simulink model "Ground"  (R2015a)
settings: configuration reference "GlobalConfig" (kept outside this file)
PreLoadFcn:
  | modelPreLoadClbck
InitFcn:
  | modelPreLoadClbck
model workspace (MAT data in the model file):
  MCOS : class17 (value not decoded)
libraries: fl_lib x427, nesl_utility x145
(part 4 of 5)

== system Ground/Ground Model 1/GroundUnit45 ==
  Conductive Heat Transfer1 : fl_lib/Thermal/Thermal Elements/Conductive Heat Transfer  area=Area m^2  thickness=Thickness/100 m  th_cond=ThermalConductivity W/(m*K)  Q_specify=off  Q_priority=High  Q=0 J/s  T_specify=off  T_priority=High  T=0 K
      settings: AttributesFormatString=|
      | Area:%<area>
      | ThCond:%<th_cond>
      | Thickness:%<thickness>
  Conductive Heat Transfer2 : fl_lib/Thermal/Thermal Elements/Conductive Heat Transfer  area=Area m^2  thickness=Thickness/100 m  th_cond=ThermalConductivity W/(m*K)  Q_specify=off  Q_priority=High  Q=0 J/s  T_specify=off  T_priority=High  T=0 K
      settings: AttributesFormatString=|
      | Area:%<area>
      | ThCond:%<th_cond>
      | Thickness:%<thickness>
  Ideal Heat Flow Sensor : fl_lib/Thermal/Thermal Sensors/Ideal Heat Flow Sensor
  Ideal Temperature Sensor : fl_lib/Thermal/Thermal Sensors/Ideal Temperature Sensor
  PS-Simulink Converter : nesl_utility/PS-Simulink Converter  PhysicalDomain=network_engine_domain  SubClassName=ps_output  LeftPortType=input  RightPortType=output  PseudoPeriodic=off  Frequencies=[]  Unit=K  AffineConversion=off
  PS-Simulink Converter1 : nesl_utility/PS-Simulink Converter  PhysicalDomain=network_engine_domain  SubClassName=ps_output  LeftPortType=input  RightPortType=output  PseudoPeriodic=off  Frequencies=[]  Unit=J/s  AffineConversion=off
  Thermal Mass : fl_lib/Thermal/Thermal Elements/Thermal Mass  mass=Density*Area*Thickness kg  sp_heat=SpecificHeat J/kg/K  Q_specify=off  Q_priority=High  Q=0 J/s  T_specify=on  T_priority=High  T=Temperature K
      settings: AttributesFormatString=|
      | %<mass>
      | %<sp_heat>
      | %<T>
  Thermal Reference1 : fl_lib/Thermal/Thermal Elements/Thermal Reference
  In : PMIOPort  Port=1  Side=Left
  Out : PMIOPort  Port=2  Side=Left
  Temperature : Outport
  Heat Flow : Outport  Port=2
  wires:
  PS-Simulink Converter/1 -> Temperature/1
  PS-Simulink Converter1/1 -> Heat Flow/1
  connections:
  Conductive Heat Transfer2/RConn1 -- Out/RConn1
  Ideal Temperature Sensor/RConn1 -- Thermal Reference1/LConn1
  Conductive Heat Transfer2/LConn1 -- Ideal Heat Flow Sensor/RConn2
  PS-Simulink Converter/LConn1 -- Ideal Temperature Sensor/RConn2
  In/RConn1 -- Conductive Heat Transfer1/LConn1
  Conductive Heat Transfer1/RConn1 -- Ideal Temperature Sensor/LConn1 -- Ideal Heat Flow Sensor/LConn1 -- Thermal Mass/LConn1
  Ideal Heat Flow Sensor/RConn1 -- PS-Simulink Converter1/LConn1

== system Ground/Ground Model 1/GroundUnit46 ==
  Conductive Heat Transfer1 : fl_lib/Thermal/Thermal Elements/Conductive Heat Transfer  area=Area m^2  thickness=Thickness/100 m  th_cond=ThermalConductivity W/(m*K)  Q_specify=off  Q_priority=High  Q=0 J/s  T_specify=off  T_priority=High  T=0 K
      settings: AttributesFormatString=|
      | Area:%<area>
      | ThCond:%<th_cond>
      | Thickness:%<thickness>
  Conductive Heat Transfer2 : fl_lib/Thermal/Thermal Elements/Conductive Heat Transfer  area=Area m^2  thickness=Thickness/100 m  th_cond=ThermalConductivity W/(m*K)  Q_specify=off  Q_priority=High  Q=0 J/s  T_specify=off  T_priority=High  T=0 K
      settings: AttributesFormatString=|
      | Area:%<area>
      | ThCond:%<th_cond>
      | Thickness:%<thickness>
  Ideal Heat Flow Sensor : fl_lib/Thermal/Thermal Sensors/Ideal Heat Flow Sensor
  Ideal Temperature Sensor : fl_lib/Thermal/Thermal Sensors/Ideal Temperature Sensor
  PS-Simulink Converter : nesl_utility/PS-Simulink Converter  PhysicalDomain=network_engine_domain  SubClassName=ps_output  LeftPortType=input  RightPortType=output  PseudoPeriodic=off  Frequencies=[]  Unit=K  AffineConversion=off
  PS-Simulink Converter1 : nesl_utility/PS-Simulink Converter  PhysicalDomain=network_engine_domain  SubClassName=ps_output  LeftPortType=input  RightPortType=output  PseudoPeriodic=off  Frequencies=[]  Unit=J/s  AffineConversion=off
  Thermal Mass : fl_lib/Thermal/Thermal Elements/Thermal Mass  mass=Density*Area*Thickness kg  sp_heat=SpecificHeat J/kg/K  Q_specify=off  Q_priority=High  Q=0 J/s  T_specify=on  T_priority=High  T=Temperature K
      settings: AttributesFormatString=|
      | %<mass>
      | %<sp_heat>
      | %<T>
  Thermal Reference1 : fl_lib/Thermal/Thermal Elements/Thermal Reference
  In : PMIOPort  Port=1  Side=Left
  Out : PMIOPort  Port=2  Side=Left
  Temperature : Outport
  Heat Flow : Outport  Port=2
  wires:
  PS-Simulink Converter/1 -> Temperature/1
  PS-Simulink Converter1/1 -> Heat Flow/1
  connections:
  Conductive Heat Transfer2/RConn1 -- Out/RConn1
  Ideal Temperature Sensor/RConn1 -- Thermal Reference1/LConn1
  Conductive Heat Transfer2/LConn1 -- Ideal Heat Flow Sensor/RConn2
  PS-Simulink Converter/LConn1 -- Ideal Temperature Sensor/RConn2
  In/RConn1 -- Conductive Heat Transfer1/LConn1
  Conductive Heat Transfer1/RConn1 -- Ideal Temperature Sensor/LConn1 -- Ideal Heat Flow Sensor/LConn1 -- Thermal Mass/LConn1
  Ideal Heat Flow Sensor/RConn1 -- PS-Simulink Converter1/LConn1

== system Ground/Ground Model 1/GroundUnit47 ==
  Conductive Heat Transfer1 : fl_lib/Thermal/Thermal Elements/Conductive Heat Transfer  area=Area m^2  thickness=Thickness/100 m  th_cond=ThermalConductivity W/(m*K)  Q_specify=off  Q_priority=High  Q=0 J/s  T_specify=off  T_priority=High  T=0 K
      settings: AttributesFormatString=|
      | Area:%<area>
      | ThCond:%<th_cond>
      | Thickness:%<thickness>
  Conductive Heat Transfer2 : fl_lib/Thermal/Thermal Elements/Conductive Heat Transfer  area=Area m^2  thickness=Thickness/100 m  th_cond=ThermalConductivity W/(m*K)  Q_specify=off  Q_priority=High  Q=0 J/s  T_specify=off  T_priority=High  T=0 K
      settings: AttributesFormatString=|
      | Area:%<area>
      | ThCond:%<th_cond>
      | Thickness:%<thickness>
  Ideal Heat Flow Sensor : fl_lib/Thermal/Thermal Sensors/Ideal Heat Flow Sensor
  Ideal Temperature Sensor : fl_lib/Thermal/Thermal Sensors/Ideal Temperature Sensor
  PS-Simulink Converter : nesl_utility/PS-Simulink Converter  PhysicalDomain=network_engine_domain  SubClassName=ps_output  LeftPortType=input  RightPortType=output  PseudoPeriodic=off  Frequencies=[]  Unit=K  AffineConversion=off
  PS-Simulink Converter1 : nesl_utility/PS-Simulink Converter  PhysicalDomain=network_engine_domain  SubClassName=ps_output  LeftPortType=input  RightPortType=output  PseudoPeriodic=off  Frequencies=[]  Unit=J/s  AffineConversion=off
  Thermal Mass : fl_lib/Thermal/Thermal Elements/Thermal Mass  mass=Density*Area*Thickness kg  sp_heat=SpecificHeat J/kg/K  Q_specify=off  Q_priority=High  Q=0 J/s  T_specify=on  T_priority=High  T=Temperature K
      settings: AttributesFormatString=|
      | %<mass>
      | %<sp_heat>
      | %<T>
  Thermal Reference1 : fl_lib/Thermal/Thermal Elements/Thermal Reference
  In : PMIOPort  Port=1  Side=Left
  Out : PMIOPort  Port=2  Side=Left
  Temperature : Outport
  Heat Flow : Outport  Port=2
  wires:
  PS-Simulink Converter/1 -> Temperature/1
  PS-Simulink Converter1/1 -> Heat Flow/1
  connections:
  Conductive Heat Transfer2/RConn1 -- Out/RConn1
  Ideal Temperature Sensor/RConn1 -- Thermal Reference1/LConn1
  Conductive Heat Transfer2/LConn1 -- Ideal Heat Flow Sensor/RConn2
  PS-Simulink Converter/LConn1 -- Ideal Temperature Sensor/RConn2
  In/RConn1 -- Conductive Heat Transfer1/LConn1
  Conductive Heat Transfer1/RConn1 -- Ideal Temperature Sensor/LConn1 -- Ideal Heat Flow Sensor/LConn1 -- Thermal Mass/LConn1
  Ideal Heat Flow Sensor/RConn1 -- PS-Simulink Converter1/LConn1

== system Ground/Ground Model 1/GroundUnit48 ==
  Conductive Heat Transfer1 : fl_lib/Thermal/Thermal Elements/Conductive Heat Transfer  area=Area m^2  thickness=Thickness/100 m  th_cond=ThermalConductivity W/(m*K)  Q_specify=off  Q_priority=High  Q=0 J/s  T_specify=off  T_priority=High  T=0 K
      settings: AttributesFormatString=|
      | Area:%<area>
      | ThCond:%<th_cond>
      | Thickness:%<thickness>
  Conductive Heat Transfer2 : fl_lib/Thermal/Thermal Elements/Conductive Heat Transfer  area=Area m^2  thickness=Thickness/100 m  th_cond=ThermalConductivity W/(m*K)  Q_specify=off  Q_priority=High  Q=0 J/s  T_specify=off  T_priority=High  T=0 K
      settings: AttributesFormatString=|
      | Area:%<area>
      | ThCond:%<th_cond>
      | Thickness:%<thickness>
  Ideal Heat Flow Sensor : fl_lib/Thermal/Thermal Sensors/Ideal Heat Flow Sensor
  Ideal Temperature Sensor : fl_lib/Thermal/Thermal Sensors/Ideal Temperature Sensor
  PS-Simulink Converter : nesl_utility/PS-Simulink Converter  PhysicalDomain=network_engine_domain  SubClassName=ps_output  LeftPortType=input  RightPortType=output  PseudoPeriodic=off  Frequencies=[]  Unit=K  AffineConversion=off
  PS-Simulink Converter1 : nesl_utility/PS-Simulink Converter  PhysicalDomain=network_engine_domain  SubClassName=ps_output  LeftPortType=input  RightPortType=output  PseudoPeriodic=off  Frequencies=[]  Unit=J/s  AffineConversion=off
  Thermal Mass : fl_lib/Thermal/Thermal Elements/Thermal Mass  mass=Density*Area*Thickness kg  sp_heat=SpecificHeat J/kg/K  Q_specify=off  Q_priority=High  Q=0 J/s  T_specify=on  T_priority=High  T=Temperature K
      settings: AttributesFormatString=|
      | %<mass>
      | %<sp_heat>
      | %<T>
  Thermal Reference1 : fl_lib/Thermal/Thermal Elements/Thermal Reference
  In : PMIOPort  Port=1  Side=Left
  Out : PMIOPort  Port=2  Side=Left
  Temperature : Outport
  Heat Flow : Outport  Port=2
  wires:
  PS-Simulink Converter/1 -> Temperature/1
  PS-Simulink Converter1/1 -> Heat Flow/1
  connections:
  Conductive Heat Transfer2/RConn1 -- Out/RConn1
  Ideal Temperature Sensor/RConn1 -- Thermal Reference1/LConn1
  Conductive Heat Transfer2/LConn1 -- Ideal Heat Flow Sensor/RConn2
  PS-Simulink Converter/LConn1 -- Ideal Temperature Sensor/RConn2
  In/RConn1 -- Conductive Heat Transfer1/LConn1
  Conductive Heat Transfer1/RConn1 -- Ideal Temperature Sensor/LConn1 -- Ideal Heat Flow Sensor/LConn1 -- Thermal Mass/LConn1
  Ideal Heat Flow Sensor/RConn1 -- PS-Simulink Converter1/LConn1

== system Ground/Ground Model 1/GroundUnit49 ==
  Conductive Heat Transfer1 : fl_lib/Thermal/Thermal Elements/Conductive Heat Transfer  area=Area m^2  thickness=Thickness/100 m  th_cond=ThermalConductivity W/(m*K)  Q_specify=off  Q_priority=High  Q=0 J/s  T_specify=off  T_priority=High  T=0 K
      settings: AttributesFormatString=|
      | Area:%<area>
      | ThCond:%<th_cond>
      | Thickness:%<thickness>
  Conductive Heat Transfer2 : fl_lib/Thermal/Thermal Elements/Conductive Heat Transfer  area=Area m^2  thickness=Thickness/100 m  th_cond=ThermalConductivity W/(m*K)  Q_specify=off  Q_priority=High  Q=0 J/s  T_specify=off  T_priority=High  T=0 K
      settings: AttributesFormatString=|
      | Area:%<area>
      | ThCond:%<th_cond>
      | Thickness:%<thickness>
  Ideal Heat Flow Sensor : fl_lib/Thermal/Thermal Sensors/Ideal Heat Flow Sensor
  Ideal Temperature Sensor : fl_lib/Thermal/Thermal Sensors/Ideal Temperature Sensor
  PS-Simulink Converter : nesl_utility/PS-Simulink Converter  PhysicalDomain=network_engine_domain  SubClassName=ps_output  LeftPortType=input  RightPortType=output  PseudoPeriodic=off  Frequencies=[]  Unit=K  AffineConversion=off
  PS-Simulink Converter1 : nesl_utility/PS-Simulink Converter  PhysicalDomain=network_engine_domain  SubClassName=ps_output  LeftPortType=input  RightPortType=output  PseudoPeriodic=off  Frequencies=[]  Unit=J/s  AffineConversion=off
  Thermal Mass : fl_lib/Thermal/Thermal Elements/Thermal Mass  mass=Density*Area*Thickness kg  sp_heat=SpecificHeat J/kg/K  Q_specify=off  Q_priority=High  Q=0 J/s  T_specify=on  T_priority=High  T=Temperature K
      settings: AttributesFormatString=|
      | %<mass>
      | %<sp_heat>
      | %<T>
  Thermal Reference1 : fl_lib/Thermal/Thermal Elements/Thermal Reference
  In : PMIOPort  Port=1  Side=Left
  Out : PMIOPort  Port=2  Side=Left
  Temperature : Outport
  Heat Flow : Outport  Port=2
  wires:
  PS-Simulink Converter/1 -> Temperature/1
  PS-Simulink Converter1/1 -> Heat Flow/1
  connections:
  Conductive Heat Transfer2/RConn1 -- Out/RConn1
  Ideal Temperature Sensor/RConn1 -- Thermal Reference1/LConn1
  Conductive Heat Transfer2/LConn1 -- Ideal Heat Flow Sensor/RConn2
  PS-Simulink Converter/LConn1 -- Ideal Temperature Sensor/RConn2
  In/RConn1 -- Conductive Heat Transfer1/LConn1
  Conductive Heat Transfer1/RConn1 -- Ideal Temperature Sensor/LConn1 -- Ideal Heat Flow Sensor/LConn1 -- Thermal Mass/LConn1
  Ideal Heat Flow Sensor/RConn1 -- PS-Simulink Converter1/LConn1

== system Ground/Ground Model 1/GroundUnit5 ==
  Conductive Heat Transfer1 : fl_lib/Thermal/Thermal Elements/Conductive Heat Transfer  area=Area m^2  thickness=Thickness/100 m  th_cond=ThermalConductivity W/(m*K)  Q_specify=off  Q_priority=High  Q=0 J/s  T_specify=off  T_priority=High  T=0 K
      settings: AttributesFormatString=|
      | Area:%<area>
      | ThCond:%<th_cond>
      | Thickness:%<thickness>
  Conductive Heat Transfer2 : fl_lib/Thermal/Thermal Elements/Conductive Heat Transfer  area=Area m^2  thickness=Thickness/100 m  th_cond=ThermalConductivity W/(m*K)  Q_specify=off  Q_priority=High  Q=0 J/s  T_specify=off  T_priority=High  T=0 K
      settings: AttributesFormatString=|
      | Area:%<area>
      | ThCond:%<th_cond>
      | Thickness:%<thickness>
  Ideal Heat Flow Sensor : fl_lib/Thermal/Thermal Sensors/Ideal Heat Flow Sensor
  Ideal Temperature Sensor : fl_lib/Thermal/Thermal Sensors/Ideal Temperature Sensor
  PS-Simulink Converter : nesl_utility/PS-Simulink Converter  PhysicalDomain=network_engine_domain  SubClassName=ps_output  LeftPortType=input  RightPortType=output  PseudoPeriodic=off  Frequencies=[]  Unit=K  AffineConversion=off
  PS-Simulink Converter1 : nesl_utility/PS-Simulink Converter  PhysicalDomain=network_engine_domain  SubClassName=ps_output  LeftPortType=input  RightPortType=output  PseudoPeriodic=off  Frequencies=[]  Unit=J/s  AffineConversion=off
  Thermal Mass : fl_lib/Thermal/Thermal Elements/Thermal Mass  mass=Density*Area*Thickness kg  sp_heat=SpecificHeat J/kg/K  Q_specify=off  Q_priority=High  Q=0 J/s  T_specify=on  T_priority=High  T=Temperature K
      settings: AttributesFormatString=|
      | %<mass>
      | %<sp_heat>
      | %<T>
  Thermal Reference1 : fl_lib/Thermal/Thermal Elements/Thermal Reference
  In : PMIOPort  Port=1  Side=Left
  Out : PMIOPort  Port=2  Side=Left
  Temperature : Outport
  Heat Flow : Outport  Port=2
  wires:
  PS-Simulink Converter/1 -> Temperature/1
  PS-Simulink Converter1/1 -> Heat Flow/1
  connections:
  Conductive Heat Transfer2/RConn1 -- Out/RConn1
  Ideal Temperature Sensor/RConn1 -- Thermal Reference1/LConn1
  Conductive Heat Transfer2/LConn1 -- Ideal Heat Flow Sensor/RConn2
  PS-Simulink Converter/LConn1 -- Ideal Temperature Sensor/RConn2
  In/RConn1 -- Conductive Heat Transfer1/LConn1
  Conductive Heat Transfer1/RConn1 -- Ideal Temperature Sensor/LConn1 -- Ideal Heat Flow Sensor/LConn1 -- Thermal Mass/LConn1
  Ideal Heat Flow Sensor/RConn1 -- PS-Simulink Converter1/LConn1

== system Ground/Ground Model 1/GroundUnit6 ==
  Conductive Heat Transfer1 : fl_lib/Thermal/Thermal Elements/Conductive Heat Transfer  area=Area m^2  thickness=Thickness/100 m  th_cond=ThermalConductivity W/(m*K)  Q_specify=off  Q_priority=High  Q=0 J/s  T_specify=off  T_priority=High  T=0 K
      settings: AttributesFormatString=|
      | Area:%<area>
      | ThCond:%<th_cond>
      | Thickness:%<thickness>
  Conductive Heat Transfer2 : fl_lib/Thermal/Thermal Elements/Conductive Heat Transfer  area=Area m^2  thickness=Thickness/100 m  th_cond=ThermalConductivity W/(m*K)  Q_specify=off  Q_priority=High  Q=0 J/s  T_specify=off  T_priority=High  T=0 K
      settings: AttributesFormatString=|
      | Area:%<area>
      | ThCond:%<th_cond>
      | Thickness:%<thickness>
  Ideal Heat Flow Sensor : fl_lib/Thermal/Thermal Sensors/Ideal Heat Flow Sensor
  Ideal Temperature Sensor : fl_lib/Thermal/Thermal Sensors/Ideal Temperature Sensor
  PS-Simulink Converter : nesl_utility/PS-Simulink Converter  PhysicalDomain=network_engine_domain  SubClassName=ps_output  LeftPortType=input  RightPortType=output  PseudoPeriodic=off  Frequencies=[]  Unit=K  AffineConversion=off
  PS-Simulink Converter1 : nesl_utility/PS-Simulink Converter  PhysicalDomain=network_engine_domain  SubClassName=ps_output  LeftPortType=input  RightPortType=output  PseudoPeriodic=off  Frequencies=[]  Unit=J/s  AffineConversion=off
  Thermal Mass : fl_lib/Thermal/Thermal Elements/Thermal Mass  mass=Density*Area*Thickness kg  sp_heat=SpecificHeat J/kg/K  Q_specify=off  Q_priority=High  Q=0 J/s  T_specify=on  T_priority=High  T=Temperature K
      settings: AttributesFormatString=|
      | %<mass>
      | %<sp_heat>
      | %<T>
  Thermal Reference1 : fl_lib/Thermal/Thermal Elements/Thermal Reference
  In : PMIOPort  Port=1  Side=Left
  Out : PMIOPort  Port=2  Side=Left
  Temperature : Outport
  Heat Flow : Outport  Port=2
  wires:
  PS-Simulink Converter/1 -> Temperature/1
  PS-Simulink Converter1/1 -> Heat Flow/1
  connections:
  Conductive Heat Transfer2/RConn1 -- Out/RConn1
  Ideal Temperature Sensor/RConn1 -- Thermal Reference1/LConn1
  Conductive Heat Transfer2/LConn1 -- Ideal Heat Flow Sensor/RConn2
  PS-Simulink Converter/LConn1 -- Ideal Temperature Sensor/RConn2
  In/RConn1 -- Conductive Heat Transfer1/LConn1
  Conductive Heat Transfer1/RConn1 -- Ideal Temperature Sensor/LConn1 -- Ideal Heat Flow Sensor/LConn1 -- Thermal Mass/LConn1
  Ideal Heat Flow Sensor/RConn1 -- PS-Simulink Converter1/LConn1

== system Ground/Ground Model 1/GroundUnit7 ==
  Conductive Heat Transfer1 : fl_lib/Thermal/Thermal Elements/Conductive Heat Transfer  area=Area m^2  thickness=Thickness/100 m  th_cond=ThermalConductivity W/(m*K)  Q_specify=off  Q_priority=High  Q=0 J/s  T_specify=off  T_priority=High  T=0 K
      settings: AttributesFormatString=|
      | Area:%<area>
      | ThCond:%<th_cond>
      | Thickness:%<thickness>
  Conductive Heat Transfer2 : fl_lib/Thermal/Thermal Elements/Conductive Heat Transfer  area=Area m^2  thickness=Thickness/100 m  th_cond=ThermalConductivity W/(m*K)  Q_specify=off  Q_priority=High  Q=0 J/s  T_specify=off  T_priority=High  T=0 K
      settings: AttributesFormatString=|
      | Area:%<area>
      | ThCond:%<th_cond>
      | Thickness:%<thickness>
  Ideal Heat Flow Sensor : fl_lib/Thermal/Thermal Sensors/Ideal Heat Flow Sensor
  Ideal Temperature Sensor : fl_lib/Thermal/Thermal Sensors/Ideal Temperature Sensor
  PS-Simulink Converter : nesl_utility/PS-Simulink Converter  PhysicalDomain=network_engine_domain  SubClassName=ps_output  LeftPortType=input  RightPortType=output  PseudoPeriodic=off  Frequencies=[]  Unit=K  AffineConversion=off
  PS-Simulink Converter1 : nesl_utility/PS-Simulink Converter  PhysicalDomain=network_engine_domain  SubClassName=ps_output  LeftPortType=input  RightPortType=output  PseudoPeriodic=off  Frequencies=[]  Unit=J/s  AffineConversion=off
  Thermal Mass : fl_lib/Thermal/Thermal Elements/Thermal Mass  mass=Density*Area*Thickness kg  sp_heat=SpecificHeat J/kg/K  Q_specify=off  Q_priority=High  Q=0 J/s  T_specify=on  T_priority=High  T=Temperature K
      settings: AttributesFormatString=|
      | %<mass>
      | %<sp_heat>
      | %<T>
  Thermal Reference1 : fl_lib/Thermal/Thermal Elements/Thermal Reference
  In : PMIOPort  Port=1  Side=Left
  Out : PMIOPort  Port=2  Side=Left
  Temperature : Outport
  Heat Flow : Outport  Port=2
  wires:
  PS-Simulink Converter/1 -> Temperature/1
  PS-Simulink Converter1/1 -> Heat Flow/1
  connections:
  Conductive Heat Transfer2/RConn1 -- Out/RConn1
  Ideal Temperature Sensor/RConn1 -- Thermal Reference1/LConn1
  Conductive Heat Transfer2/LConn1 -- Ideal Heat Flow Sensor/RConn2
  PS-Simulink Converter/LConn1 -- Ideal Temperature Sensor/RConn2
  In/RConn1 -- Conductive Heat Transfer1/LConn1
  Conductive Heat Transfer1/RConn1 -- Ideal Temperature Sensor/LConn1 -- Ideal Heat Flow Sensor/LConn1 -- Thermal Mass/LConn1
  Ideal Heat Flow Sensor/RConn1 -- PS-Simulink Converter1/LConn1

== system Ground/Ground Model 1/GroundUnit8 ==
  Conductive Heat Transfer1 : fl_lib/Thermal/Thermal Elements/Conductive Heat Transfer  area=Area m^2  thickness=Thickness/100 m  th_cond=ThermalConductivity W/(m*K)  Q_specify=off  Q_priority=High  Q=0 J/s  T_specify=off  T_priority=High  T=0 K
      settings: AttributesFormatString=|
      | Area:%<area>
      | ThCond:%<th_cond>
      | Thickness:%<thickness>
  Conductive Heat Transfer2 : fl_lib/Thermal/Thermal Elements/Conductive Heat Transfer  area=Area m^2  thickness=Thickness/100 m  th_cond=ThermalConductivity W/(m*K)  Q_specify=off  Q_priority=High  Q=0 J/s  T_specify=off  T_priority=High  T=0 K
      settings: AttributesFormatString=|
      | Area:%<area>
      | ThCond:%<th_cond>
      | Thickness:%<thickness>
  Ideal Heat Flow Sensor : fl_lib/Thermal/Thermal Sensors/Ideal Heat Flow Sensor
  Ideal Temperature Sensor : fl_lib/Thermal/Thermal Sensors/Ideal Temperature Sensor
  PS-Simulink Converter : nesl_utility/PS-Simulink Converter  PhysicalDomain=network_engine_domain  SubClassName=ps_output  LeftPortType=input  RightPortType=output  PseudoPeriodic=off  Frequencies=[]  Unit=K  AffineConversion=off
  PS-Simulink Converter1 : nesl_utility/PS-Simulink Converter  PhysicalDomain=network_engine_domain  SubClassName=ps_output  LeftPortType=input  RightPortType=output  PseudoPeriodic=off  Frequencies=[]  Unit=J/s  AffineConversion=off
  Thermal Mass : fl_lib/Thermal/Thermal Elements/Thermal Mass  mass=Density*Area*Thickness kg  sp_heat=SpecificHeat J/kg/K  Q_specify=off  Q_priority=High  Q=0 J/s  T_specify=on  T_priority=High  T=Temperature K
      settings: AttributesFormatString=|
      | %<mass>
      | %<sp_heat>
      | %<T>
  Thermal Reference1 : fl_lib/Thermal/Thermal Elements/Thermal Reference
  In : PMIOPort  Port=1  Side=Left
  Out : PMIOPort  Port=2  Side=Left
  Temperature : Outport
  Heat Flow : Outport  Port=2
  wires:
  PS-Simulink Converter/1 -> Temperature/1
  PS-Simulink Converter1/1 -> Heat Flow/1
  connections:
  Conductive Heat Transfer2/RConn1 -- Out/RConn1
  Ideal Temperature Sensor/RConn1 -- Thermal Reference1/LConn1
  Conductive Heat Transfer2/LConn1 -- Ideal Heat Flow Sensor/RConn2
  PS-Simulink Converter/LConn1 -- Ideal Temperature Sensor/RConn2
  In/RConn1 -- Conductive Heat Transfer1/LConn1
  Conductive Heat Transfer1/RConn1 -- Ideal Temperature Sensor/LConn1 -- Ideal Heat Flow Sensor/LConn1 -- Thermal Mass/LConn1
  Ideal Heat Flow Sensor/RConn1 -- PS-Simulink Converter1/LConn1

== system Ground/Ground Model 1/GroundUnit9 ==
  Conductive Heat Transfer1 : fl_lib/Thermal/Thermal Elements/Conductive Heat Transfer  area=Area m^2  thickness=Thickness/100 m  th_cond=ThermalConductivity W/(m*K)  Q_specify=off  Q_priority=High  Q=0 J/s  T_specify=off  T_priority=High  T=0 K
      settings: AttributesFormatString=|
      | Area:%<area>
      | ThCond:%<th_cond>
      | Thickness:%<thickness>
  Conductive Heat Transfer2 : fl_lib/Thermal/Thermal Elements/Conductive Heat Transfer  area=Area m^2  thickness=Thickness/100 m  th_cond=ThermalConductivity W/(m*K)  Q_specify=off  Q_priority=High  Q=0 J/s  T_specify=off  T_priority=High  T=0 K
      settings: AttributesFormatString=|
      | Area:%<area>
      | ThCond:%<th_cond>
      | Thickness:%<thickness>
  Ideal Heat Flow Sensor : fl_lib/Thermal/Thermal Sensors/Ideal Heat Flow Sensor
  Ideal Temperature Sensor : fl_lib/Thermal/Thermal Sensors/Ideal Temperature Sensor
  PS-Simulink Converter : nesl_utility/PS-Simulink Converter  PhysicalDomain=network_engine_domain  SubClassName=ps_output  LeftPortType=input  RightPortType=output  PseudoPeriodic=off  Frequencies=[]  Unit=K  AffineConversion=off
  PS-Simulink Converter1 : nesl_utility/PS-Simulink Converter  PhysicalDomain=network_engine_domain  SubClassName=ps_output  LeftPortType=input  RightPortType=output  PseudoPeriodic=off  Frequencies=[]  Unit=J/s  AffineConversion=off
  Thermal Mass : fl_lib/Thermal/Thermal Elements/Thermal Mass  mass=Density*Area*Thickness kg  sp_heat=SpecificHeat J/kg/K  Q_specify=off  Q_priority=High  Q=0 J/s  T_specify=on  T_priority=High  T=Temperature K
      settings: AttributesFormatString=|
      | %<mass>
      | %<sp_heat>
      | %<T>
  Thermal Reference1 : fl_lib/Thermal/Thermal Elements/Thermal Reference
  In : PMIOPort  Port=1  Side=Left
  Out : PMIOPort  Port=2  Side=Left
  Temperature : Outport
  Heat Flow : Outport  Port=2
  wires:
  PS-Simulink Converter/1 -> Temperature/1
  PS-Simulink Converter1/1 -> Heat Flow/1
  connections:
  Conductive Heat Transfer2/RConn1 -- Out/RConn1
  Ideal Temperature Sensor/RConn1 -- Thermal Reference1/LConn1
  Conductive Heat Transfer2/LConn1 -- Ideal Heat Flow Sensor/RConn2
  PS-Simulink Converter/LConn1 -- Ideal Temperature Sensor/RConn2
  In/RConn1 -- Conductive Heat Transfer1/LConn1
  Conductive Heat Transfer1/RConn1 -- Ideal Temperature Sensor/LConn1 -- Ideal Heat Flow Sensor/LConn1 -- Thermal Mass/LConn1
  Ideal Heat Flow Sensor/RConn1 -- PS-Simulink Converter1/LConn1

== system Ground/Ground Model 8/GroundUnit0 ==
  Conductive Heat Transfer1 : fl_lib/Thermal/Thermal Elements/Conductive Heat Transfer  area=Area m^2  thickness=Thickness/MeshNum m  th_cond=ThermalConductivity W/(m*K)  Q_specify=off  Q_priority=High  Q=0 J/s  T_specify=off  T_priority=High  T=0 K
      settings: AttributesFormatString=|
      | Area:%<area>
      | ThCond:%<th_cond>
      | Thickness:%<thickness>
  Conductive Heat Transfer2 : fl_lib/Thermal/Thermal Elements/Conductive Heat Transfer  area=Area m^2  thickness=Thickness/MeshNum m  th_cond=ThermalConductivity W/(m*K)  Q_specify=off  Q_priority=High  Q=0 J/s  T_specify=off  T_priority=High  T=0 K
      settings: AttributesFormatString=|
      | Area:%<area>
      | ThCond:%<th_cond>
      | Thickness:%<thickness>
  Ideal Heat Flow Sensor : fl_lib/Thermal/Thermal Sensors/Ideal Heat Flow Sensor
  Ideal Temperature Sensor : fl_lib/Thermal/Thermal Sensors/Ideal Temperature Sensor
  PS-Simulink Converter : nesl_utility/PS-Simulink Converter  PhysicalDomain=network_engine_domain  SubClassName=ps_output  LeftPortType=input  RightPortType=output  PseudoPeriodic=off  Frequencies=[]  Unit=K  AffineConversion=off
  PS-Simulink Converter1 : nesl_utility/PS-Simulink Converter  PhysicalDomain=network_engine_domain  SubClassName=ps_output  LeftPortType=input  RightPortType=output  PseudoPeriodic=off  Frequencies=[]  Unit=J/s  AffineConversion=off
  Terminator : Terminator
  Thermal Mass : fl_lib/Thermal/Thermal Elements/Thermal Mass  mass=Density*Area*Thickness kg  sp_heat=SpecificHeat J/kg/K  Q_specify=off  Q_priority=High  Q=0 J/s  T_specify=on  T_priority=High  T=Temperature K
      settings: AttributesFormatString=|
      | %<mass>
      | %<sp_heat>
      | %<T>
  Thermal Reference1 : fl_lib/Thermal/Thermal Elements/Thermal Reference
  In : PMIOPort  Port=1  Side=Left
  Out : PMIOPort  Port=2  Side=Left
  Temperature : Outport
  wires:
  PS-Simulink Converter/1 -> Temperature/1
  PS-Simulink Converter1/1 -> Terminator/1
  connections:
  Conductive Heat Transfer2/RConn1 -- Out/RConn1
  Ideal Temperature Sensor/RConn1 -- Thermal Reference1/LConn1
  Conductive Heat Transfer2/LConn1 -- Ideal Heat Flow Sensor/RConn2
  PS-Simulink Converter/LConn1 -- Ideal Temperature Sensor/RConn2
  In/RConn1 -- Conductive Heat Transfer1/LConn1
  Conductive Heat Transfer1/RConn1 -- Ideal Temperature Sensor/LConn1 -- Ideal Heat Flow Sensor/LConn1 -- Thermal Mass/LConn1
  Ideal Heat Flow Sensor/RConn1 -- PS-Simulink Converter1/LConn1

== system Ground/Ground Model 8/GroundUnit1 ==
  Conductive Heat Transfer1 : fl_lib/Thermal/Thermal Elements/Conductive Heat Transfer  area=Area m^2  thickness=Thickness/MeshNum m  th_cond=ThermalConductivity W/(m*K)  Q_specify=off  Q_priority=High  Q=0 J/s  T_specify=off  T_priority=High  T=0 K
      settings: AttributesFormatString=|
      | Area:%<area>
      | ThCond:%<th_cond>
      | Thickness:%<thickness>
  Conductive Heat Transfer2 : fl_lib/Thermal/Thermal Elements/Conductive Heat Transfer  area=Area m^2  thickness=Thickness/MeshNum m  th_cond=ThermalConductivity W/(m*K)  Q_specify=off  Q_priority=High  Q=0 J/s  T_specify=off  T_priority=High  T=0 K
      settings: AttributesFormatString=|
      | Area:%<area>
      | ThCond:%<th_cond>
      | Thickness:%<thickness>
  Ideal Heat Flow Sensor : fl_lib/Thermal/Thermal Sensors/Ideal Heat Flow Sensor
  Ideal Temperature Sensor : fl_lib/Thermal/Thermal Sensors/Ideal Temperature Sensor
  PS-Simulink Converter : nesl_utility/PS-Simulink Converter  PhysicalDomain=network_engine_domain  SubClassName=ps_output  LeftPortType=input  RightPortType=output  PseudoPeriodic=off  Frequencies=[]  Unit=K  AffineConversion=off
  PS-Simulink Converter1 : nesl_utility/PS-Simulink Converter  PhysicalDomain=network_engine_domain  SubClassName=ps_output  LeftPortType=input  RightPortType=output  PseudoPeriodic=off  Frequencies=[]  Unit=J/s  AffineConversion=off
  Terminator : Terminator
  Thermal Mass : fl_lib/Thermal/Thermal Elements/Thermal Mass  mass=Density*Area*Thickness kg  sp_heat=SpecificHeat J/kg/K  Q_specify=off  Q_priority=High  Q=0 J/s  T_specify=on  T_priority=High  T=Temperature K
      settings: AttributesFormatString=|
      | %<mass>
      | %<sp_heat>
      | %<T>
  Thermal Reference1 : fl_lib/Thermal/Thermal Elements/Thermal Reference
  In : PMIOPort  Port=1  Side=Left
  Out : PMIOPort  Port=2  Side=Left
  Temperature : Outport
  wires:
  PS-Simulink Converter/1 -> Temperature/1
  PS-Simulink Converter1/1 -> Terminator/1
  connections:
  Conductive Heat Transfer2/RConn1 -- Out/RConn1
  Ideal Temperature Sensor/RConn1 -- Thermal Reference1/LConn1
  Conductive Heat Transfer2/LConn1 -- Ideal Heat Flow Sensor/RConn2
  PS-Simulink Converter/LConn1 -- Ideal Temperature Sensor/RConn2
  In/RConn1 -- Conductive Heat Transfer1/LConn1
  Conductive Heat Transfer1/RConn1 -- Ideal Temperature Sensor/LConn1 -- Ideal Heat Flow Sensor/LConn1 -- Thermal Mass/LConn1
  Ideal Heat Flow Sensor/RConn1 -- PS-Simulink Converter1/LConn1

== system Ground/Ground Model 8/GroundUnit10 ==
  Conductive Heat Transfer1 : fl_lib/Thermal/Thermal Elements/Conductive Heat Transfer  area=Area m^2  thickness=Thickness/MeshNum m  th_cond=ThermalConductivity W/(m*K)  Q_specify=off  Q_priority=High  Q=0 J/s  T_specify=off  T_priority=High  T=0 K
      settings: AttributesFormatString=|
      | Area:%<area>
      | ThCond:%<th_cond>
      | Thickness:%<thickness>
  Conductive Heat Transfer2 : fl_lib/Thermal/Thermal Elements/Conductive Heat Transfer  area=Area m^2  thickness=Thickness/MeshNum m  th_cond=ThermalConductivity W/(m*K)  Q_specify=off  Q_priority=High  Q=0 J/s  T_specify=off  T_priority=High  T=0 K
      settings: AttributesFormatString=|
      | Area:%<area>
      | ThCond:%<th_cond>
      | Thickness:%<thickness>
  Ideal Heat Flow Sensor : fl_lib/Thermal/Thermal Sensors/Ideal Heat Flow Sensor
  Ideal Temperature Sensor : fl_lib/Thermal/Thermal Sensors/Ideal Temperature Sensor
  PS-Simulink Converter : nesl_utility/PS-Simulink Converter  PhysicalDomain=network_engine_domain  SubClassName=ps_output  LeftPortType=input  RightPortType=output  PseudoPeriodic=off  Frequencies=[]  Unit=K  AffineConversion=off
  PS-Simulink Converter1 : nesl_utility/PS-Simulink Converter  PhysicalDomain=network_engine_domain  SubClassName=ps_output  LeftPortType=input  RightPortType=output  PseudoPeriodic=off  Frequencies=[]  Unit=J/s  AffineConversion=off
  Terminator : Terminator
  Thermal Mass : fl_lib/Thermal/Thermal Elements/Thermal Mass  mass=Density*Area*Thickness kg  sp_heat=SpecificHeat J/kg/K  Q_specify=off  Q_priority=High  Q=0 J/s  T_specify=on  T_priority=High  T=Temperature K
      settings: AttributesFormatString=|
      | %<mass>
      | %<sp_heat>
      | %<T>
  Thermal Reference1 : fl_lib/Thermal/Thermal Elements/Thermal Reference
  In : PMIOPort  Port=1  Side=Left
  Out : PMIOPort  Port=2  Side=Left
  Temperature : Outport
  wires:
  PS-Simulink Converter/1 -> Temperature/1
  PS-Simulink Converter1/1 -> Terminator/1
  connections:
  Conductive Heat Transfer2/RConn1 -- Out/RConn1
  Ideal Temperature Sensor/RConn1 -- Thermal Reference1/LConn1
  Conductive Heat Transfer2/LConn1 -- Ideal Heat Flow Sensor/RConn2
  PS-Simulink Converter/LConn1 -- Ideal Temperature Sensor/RConn2
  In/RConn1 -- Conductive Heat Transfer1/LConn1
  Conductive Heat Transfer1/RConn1 -- Ideal Temperature Sensor/LConn1 -- Ideal Heat Flow Sensor/LConn1 -- Thermal Mass/LConn1
  Ideal Heat Flow Sensor/RConn1 -- PS-Simulink Converter1/LConn1

== system Ground/Ground Model 8/GroundUnit11 ==
  Conductive Heat Transfer1 : fl_lib/Thermal/Thermal Elements/Conductive Heat Transfer  area=Area m^2  thickness=Thickness/MeshNum m  th_cond=ThermalConductivity W/(m*K)  Q_specify=off  Q_priority=High  Q=0 J/s  T_specify=off  T_priority=High  T=0 K
      settings: AttributesFormatString=|
      | Area:%<area>
      | ThCond:%<th_cond>
      | Thickness:%<thickness>
  Conductive Heat Transfer2 : fl_lib/Thermal/Thermal Elements/Conductive Heat Transfer  area=Area m^2  thickness=Thickness/MeshNum m  th_cond=ThermalConductivity W/(m*K)  Q_specify=off  Q_priority=High  Q=0 J/s  T_specify=off  T_priority=High  T=0 K
      settings: AttributesFormatString=|
      | Area:%<area>
      | ThCond:%<th_cond>
      | Thickness:%<thickness>
  Ideal Heat Flow Sensor : fl_lib/Thermal/Thermal Sensors/Ideal Heat Flow Sensor
  Ideal Temperature Sensor : fl_lib/Thermal/Thermal Sensors/Ideal Temperature Sensor
  PS-Simulink Converter : nesl_utility/PS-Simulink Converter  PhysicalDomain=network_engine_domain  SubClassName=ps_output  LeftPortType=input  RightPortType=output  PseudoPeriodic=off  Frequencies=[]  Unit=K  AffineConversion=off
  PS-Simulink Converter1 : nesl_utility/PS-Simulink Converter  PhysicalDomain=network_engine_domain  SubClassName=ps_output  LeftPortType=input  RightPortType=output  PseudoPeriodic=off  Frequencies=[]  Unit=J/s  AffineConversion=off
  Terminator : Terminator
  Thermal Mass : fl_lib/Thermal/Thermal Elements/Thermal Mass  mass=Density*Area*Thickness kg  sp_heat=SpecificHeat J/kg/K  Q_specify=off  Q_priority=High  Q=0 J/s  T_specify=on  T_priority=High  T=Temperature K
      settings: AttributesFormatString=|
      | %<mass>
      | %<sp_heat>
      | %<T>
  Thermal Reference1 : fl_lib/Thermal/Thermal Elements/Thermal Reference
  In : PMIOPort  Port=1  Side=Left
  Out : PMIOPort  Port=2  Side=Left
  Temperature : Outport
  wires:
  PS-Simulink Converter/1 -> Temperature/1
  PS-Simulink Converter1/1 -> Terminator/1
  connections:
  Conductive Heat Transfer2/RConn1 -- Out/RConn1
  Ideal Temperature Sensor/RConn1 -- Thermal Reference1/LConn1
  Conductive Heat Transfer2/LConn1 -- Ideal Heat Flow Sensor/RConn2
  PS-Simulink Converter/LConn1 -- Ideal Temperature Sensor/RConn2
  In/RConn1 -- Conductive Heat Transfer1/LConn1
  Conductive Heat Transfer1/RConn1 -- Ideal Temperature Sensor/LConn1 -- Ideal Heat Flow Sensor/LConn1 -- Thermal Mass/LConn1
  Ideal Heat Flow Sensor/RConn1 -- PS-Simulink Converter1/LConn1

== system Ground/Ground Model 8/GroundUnit12 ==
  Conductive Heat Transfer1 : fl_lib/Thermal/Thermal Elements/Conductive Heat Transfer  area=Area m^2  thickness=Thickness/MeshNum m  th_cond=ThermalConductivity W/(m*K)  Q_specify=off  Q_priority=High  Q=0 J/s  T_specify=off  T_priority=High  T=0 K
      settings: AttributesFormatString=|
      | Area:%<area>
      | ThCond:%<th_cond>
      | Thickness:%<thickness>
  Conductive Heat Transfer2 : fl_lib/Thermal/Thermal Elements/Conductive Heat Transfer  area=Area m^2  thickness=Thickness/MeshNum m  th_cond=ThermalConductivity W/(m*K)  Q_specify=off  Q_priority=High  Q=0 J/s  T_specify=off  T_priority=High  T=0 K
      settings: AttributesFormatString=|
      | Area:%<area>
      | ThCond:%<th_cond>
      | Thickness:%<thickness>
  Ideal Heat Flow Sensor : fl_lib/Thermal/Thermal Sensors/Ideal Heat Flow Sensor
  Ideal Temperature Sensor : fl_lib/Thermal/Thermal Sensors/Ideal Temperature Sensor
  PS-Simulink Converter : nesl_utility/PS-Simulink Converter  PhysicalDomain=network_engine_domain  SubClassName=ps_output  LeftPortType=input  RightPortType=output  PseudoPeriodic=off  Frequencies=[]  Unit=K  AffineConversion=off
  PS-Simulink Converter1 : nesl_utility/PS-Simulink Converter  PhysicalDomain=network_engine_domain  SubClassName=ps_output  LeftPortType=input  RightPortType=output  PseudoPeriodic=off  Frequencies=[]  Unit=J/s  AffineConversion=off
  Terminator : Terminator
  Thermal Mass : fl_lib/Thermal/Thermal Elements/Thermal Mass  mass=Density*Area*Thickness kg  sp_heat=SpecificHeat J/kg/K  Q_specify=off  Q_priority=High  Q=0 J/s  T_specify=on  T_priority=High  T=Temperature K
      settings: AttributesFormatString=|
      | %<mass>
      | %<sp_heat>
      | %<T>
  Thermal Reference1 : fl_lib/Thermal/Thermal Elements/Thermal Reference
  In : PMIOPort  Port=1  Side=Left
  Out : PMIOPort  Port=2  Side=Left
  Temperature : Outport
  wires:
  PS-Simulink Converter/1 -> Temperature/1
  PS-Simulink Converter1/1 -> Terminator/1
  connections:
  Conductive Heat Transfer2/RConn1 -- Out/RConn1
  Ideal Temperature Sensor/RConn1 -- Thermal Reference1/LConn1
  Conductive Heat Transfer2/LConn1 -- Ideal Heat Flow Sensor/RConn2
  PS-Simulink Converter/LConn1 -- Ideal Temperature Sensor/RConn2
  In/RConn1 -- Conductive Heat Transfer1/LConn1
  Conductive Heat Transfer1/RConn1 -- Ideal Temperature Sensor/LConn1 -- Ideal Heat Flow Sensor/LConn1 -- Thermal Mass/LConn1
  Ideal Heat Flow Sensor/RConn1 -- PS-Simulink Converter1/LConn1

== system Ground/Ground Model 8/GroundUnit13 ==
  Conductive Heat Transfer1 : fl_lib/Thermal/Thermal Elements/Conductive Heat Transfer  area=Area m^2  thickness=Thickness/MeshNum m  th_cond=ThermalConductivity W/(m*K)  Q_specify=off  Q_priority=High  Q=0 J/s  T_specify=off  T_priority=High  T=0 K
      settings: AttributesFormatString=|
      | Area:%<area>
      | ThCond:%<th_cond>
      | Thickness:%<thickness>
  Conductive Heat Transfer2 : fl_lib/Thermal/Thermal Elements/Conductive Heat Transfer  area=Area m^2  thickness=Thickness/MeshNum m  th_cond=ThermalConductivity W/(m*K)  Q_specify=off  Q_priority=High  Q=0 J/s  T_specify=off  T_priority=High  T=0 K
      settings: AttributesFormatString=|
      | Area:%<area>
      | ThCond:%<th_cond>
      | Thickness:%<thickness>
  Ideal Heat Flow Sensor : fl_lib/Thermal/Thermal Sensors/Ideal Heat Flow Sensor
  Ideal Temperature Sensor : fl_lib/Thermal/Thermal Sensors/Ideal Temperature Sensor
  PS-Simulink Converter : nesl_utility/PS-Simulink Converter  PhysicalDomain=network_engine_domain  SubClassName=ps_output  LeftPortType=input  RightPortType=output  PseudoPeriodic=off  Frequencies=[]  Unit=K  AffineConversion=off
  PS-Simulink Converter1 : nesl_utility/PS-Simulink Converter  PhysicalDomain=network_engine_domain  SubClassName=ps_output  LeftPortType=input  RightPortType=output  PseudoPeriodic=off  Frequencies=[]  Unit=J/s  AffineConversion=off
  Terminator : Terminator
  Thermal Mass : fl_lib/Thermal/Thermal Elements/Thermal Mass  mass=Density*Area*Thickness kg  sp_heat=SpecificHeat J/kg/K  Q_specify=off  Q_priority=High  Q=0 J/s  T_specify=on  T_priority=High  T=Temperature K
      settings: AttributesFormatString=|
      | %<mass>
      | %<sp_heat>
      | %<T>
  Thermal Reference1 : fl_lib/Thermal/Thermal Elements/Thermal Reference
  In : PMIOPort  Port=1  Side=Left
  Out : PMIOPort  Port=2  Side=Left
  Temperature : Outport
  wires:
  PS-Simulink Converter/1 -> Temperature/1
  PS-Simulink Converter1/1 -> Terminator/1
  connections:
  Conductive Heat Transfer2/RConn1 -- Out/RConn1
  Ideal Temperature Sensor/RConn1 -- Thermal Reference1/LConn1
  Conductive Heat Transfer2/LConn1 -- Ideal Heat Flow Sensor/RConn2
  PS-Simulink Converter/LConn1 -- Ideal Temperature Sensor/RConn2
  In/RConn1 -- Conductive Heat Transfer1/LConn1
  Conductive Heat Transfer1/RConn1 -- Ideal Temperature Sensor/LConn1 -- Ideal Heat Flow Sensor/LConn1 -- Thermal Mass/LConn1
  Ideal Heat Flow Sensor/RConn1 -- PS-Simulink Converter1/LConn1

== system Ground/Ground Model 8/GroundUnit14 ==
  Conductive Heat Transfer1 : fl_lib/Thermal/Thermal Elements/Conductive Heat Transfer  area=Area m^2  thickness=Thickness/MeshNum m  th_cond=ThermalConductivity W/(m*K)  Q_specify=off  Q_priority=High  Q=0 J/s  T_specify=off  T_priority=High  T=0 K
      settings: AttributesFormatString=|
      | Area:%<area>
      | ThCond:%<th_cond>
      | Thickness:%<thickness>
  Conductive Heat Transfer2 : fl_lib/Thermal/Thermal Elements/Conductive Heat Transfer  area=Area m^2  thickness=Thickness/MeshNum m  th_cond=ThermalConductivity W/(m*K)  Q_specify=off  Q_priority=High  Q=0 J/s  T_specify=off  T_priority=High  T=0 K
      settings: AttributesFormatString=|
      | Area:%<area>
      | ThCond:%<th_cond>
      | Thickness:%<thickness>
  Ideal Heat Flow Sensor : fl_lib/Thermal/Thermal Sensors/Ideal Heat Flow Sensor
  Ideal Temperature Sensor : fl_lib/Thermal/Thermal Sensors/Ideal Temperature Sensor
  PS-Simulink Converter : nesl_utility/PS-Simulink Converter  PhysicalDomain=network_engine_domain  SubClassName=ps_output  LeftPortType=input  RightPortType=output  PseudoPeriodic=off  Frequencies=[]  Unit=K  AffineConversion=off
  PS-Simulink Converter1 : nesl_utility/PS-Simulink Converter  PhysicalDomain=network_engine_domain  SubClassName=ps_output  LeftPortType=input  RightPortType=output  PseudoPeriodic=off  Frequencies=[]  Unit=J/s  AffineConversion=off
  Terminator : Terminator
  Thermal Mass : fl_lib/Thermal/Thermal Elements/Thermal Mass  mass=Density*Area*Thickness kg  sp_heat=SpecificHeat J/kg/K  Q_specify=off  Q_priority=High  Q=0 J/s  T_specify=on  T_priority=High  T=Temperature K
      settings: AttributesFormatString=|
      | %<mass>
      | %<sp_heat>
      | %<T>
  Thermal Reference1 : fl_lib/Thermal/Thermal Elements/Thermal Reference
  In : PMIOPort  Port=1  Side=Left
  Out : PMIOPort  Port=2  Side=Left
  Temperature : Outport
  wires:
  PS-Simulink Converter/1 -> Temperature/1
  PS-Simulink Converter1/1 -> Terminator/1
  connections:
  Conductive Heat Transfer2/RConn1 -- Out/RConn1
  Ideal Temperature Sensor/RConn1 -- Thermal Reference1/LConn1
  Conductive Heat Transfer2/LConn1 -- Ideal Heat Flow Sensor/RConn2
  PS-Simulink Converter/LConn1 -- Ideal Temperature Sensor/RConn2
  In/RConn1 -- Conductive Heat Transfer1/LConn1
  Conductive Heat Transfer1/RConn1 -- Ideal Temperature Sensor/LConn1 -- Ideal Heat Flow Sensor/LConn1 -- Thermal Mass/LConn1
  Ideal Heat Flow Sensor/RConn1 -- PS-Simulink Converter1/LConn1

== system Ground/Ground Model 8/GroundUnit15 ==
  Conductive Heat Transfer1 : fl_lib/Thermal/Thermal Elements/Conductive Heat Transfer  area=Area m^2  thickness=Thickness/MeshNum m  th_cond=ThermalConductivity W/(m*K)  Q_specify=off  Q_priority=High  Q=0 J/s  T_specify=off  T_priority=High  T=0 K
      settings: AttributesFormatString=|
      | Area:%<area>
      | ThCond:%<th_cond>
      | Thickness:%<thickness>
  Conductive Heat Transfer2 : fl_lib/Thermal/Thermal Elements/Conductive Heat Transfer  area=Area m^2  thickness=Thickness/MeshNum m  th_cond=ThermalConductivity W/(m*K)  Q_specify=off  Q_priority=High  Q=0 J/s  T_specify=off  T_priority=High  T=0 K
      settings: AttributesFormatString=|
      | Area:%<area>
      | ThCond:%<th_cond>
      | Thickness:%<thickness>
  Ideal Heat Flow Sensor : fl_lib/Thermal/Thermal Sensors/Ideal Heat Flow Sensor
  Ideal Temperature Sensor : fl_lib/Thermal/Thermal Sensors/Ideal Temperature Sensor
  PS-Simulink Converter : nesl_utility/PS-Simulink Converter  PhysicalDomain=network_engine_domain  SubClassName=ps_output  LeftPortType=input  RightPortType=output  PseudoPeriodic=off  Frequencies=[]  Unit=K  AffineConversion=off
  PS-Simulink Converter1 : nesl_utility/PS-Simulink Converter  PhysicalDomain=network_engine_domain  SubClassName=ps_output  LeftPortType=input  RightPortType=output  PseudoPeriodic=off  Frequencies=[]  Unit=J/s  AffineConversion=off
  Terminator : Terminator
  Thermal Mass : fl_lib/Thermal/Thermal Elements/Thermal Mass  mass=Density*Area*Thickness kg  sp_heat=SpecificHeat J/kg/K  Q_specify=off  Q_priority=High  Q=0 J/s  T_specify=on  T_priority=High  T=Temperature K
      settings: AttributesFormatString=|
      | %<mass>
      | %<sp_heat>
      | %<T>
  Thermal Reference1 : fl_lib/Thermal/Thermal Elements/Thermal Reference
  In : PMIOPort  Port=1  Side=Left
  Out : PMIOPort  Port=2  Side=Left
  Temperature : Outport
  wires:
  PS-Simulink Converter/1 -> Temperature/1
  PS-Simulink Converter1/1 -> Terminator/1
  connections:
  Conductive Heat Transfer2/RConn1 -- Out/RConn1
  Ideal Temperature Sensor/RConn1 -- Thermal Reference1/LConn1
  Conductive Heat Transfer2/LConn1 -- Ideal Heat Flow Sensor/RConn2
  PS-Simulink Converter/LConn1 -- Ideal Temperature Sensor/RConn2
  In/RConn1 -- Conductive Heat Transfer1/LConn1
  Conductive Heat Transfer1/RConn1 -- Ideal Temperature Sensor/LConn1 -- Ideal Heat Flow Sensor/LConn1 -- Thermal Mass/LConn1
  Ideal Heat Flow Sensor/RConn1 -- PS-Simulink Converter1/LConn1

== system Ground/Ground Model 8/GroundUnit16 ==
  Conductive Heat Transfer1 : fl_lib/Thermal/Thermal Elements/Conductive Heat Transfer  area=Area m^2  thickness=Thickness/MeshNum m  th_cond=ThermalConductivity W/(m*K)  Q_specify=off  Q_priority=High  Q=0 J/s  T_specify=off  T_priority=High  T=0 K
      settings: AttributesFormatString=|
      | Area:%<area>
      | ThCond:%<th_cond>
      | Thickness:%<thickness>
  Conductive Heat Transfer2 : fl_lib/Thermal/Thermal Elements/Conductive Heat Transfer  area=Area m^2  thickness=Thickness/MeshNum m  th_cond=ThermalConductivity W/(m*K)  Q_specify=off  Q_priority=High  Q=0 J/s  T_specify=off  T_priority=High  T=0 K
      settings: AttributesFormatString=|
      | Area:%<area>
      | ThCond:%<th_cond>
      | Thickness:%<thickness>
  Ideal Heat Flow Sensor : fl_lib/Thermal/Thermal Sensors/Ideal Heat Flow Sensor
  Ideal Temperature Sensor : fl_lib/Thermal/Thermal Sensors/Ideal Temperature Sensor
  PS-Simulink Converter : nesl_utility/PS-Simulink Converter  PhysicalDomain=network_engine_domain  SubClassName=ps_output  LeftPortType=input  RightPortType=output  PseudoPeriodic=off  Frequencies=[]  Unit=K  AffineConversion=off
  PS-Simulink Converter1 : nesl_utility/PS-Simulink Converter  PhysicalDomain=network_engine_domain  SubClassName=ps_output  LeftPortType=input  RightPortType=output  PseudoPeriodic=off  Frequencies=[]  Unit=J/s  AffineConversion=off
  Terminator : Terminator
  Thermal Mass : fl_lib/Thermal/Thermal Elements/Thermal Mass  mass=Density*Area*Thickness kg  sp_heat=SpecificHeat J/kg/K  Q_specify=off  Q_priority=High  Q=0 J/s  T_specify=on  T_priority=High  T=Temperature K
      settings: AttributesFormatString=|
      | %<mass>
      | %<sp_heat>
      | %<T>
  Thermal Reference1 : fl_lib/Thermal/Thermal Elements/Thermal Reference
  In : PMIOPort  Port=1  Side=Left
  Out : PMIOPort  Port=2  Side=Left
  Temperature : Outport
  wires:
  PS-Simulink Converter/1 -> Temperature/1
  PS-Simulink Converter1/1 -> Terminator/1
  connections:
  Conductive Heat Transfer2/RConn1 -- Out/RConn1
  Ideal Temperature Sensor/RConn1 -- Thermal Reference1/LConn1
  Conductive Heat Transfer2/LConn1 -- Ideal Heat Flow Sensor/RConn2
  PS-Simulink Converter/LConn1 -- Ideal Temperature Sensor/RConn2
  In/RConn1 -- Conductive Heat Transfer1/LConn1
  Conductive Heat Transfer1/RConn1 -- Ideal Temperature Sensor/LConn1 -- Ideal Heat Flow Sensor/LConn1 -- Thermal Mass/LConn1
  Ideal Heat Flow Sensor/RConn1 -- PS-Simulink Converter1/LConn1
